simulink model "comm_test_server_OA"  (R2014a)
settings: Solver=ode4  StartTime=0.0  StopTime=inf  FixedStep=0.01  RelTol=1e-3
libraries: SimulinkExecutionControl x1
settings Model: Creator=Tulga Ersal  LastModifiedBy=zhengys
settings OptimizationCC: ExpressionDepthLimit=2147483647
settings DebuggingCC: UnderspecifiedInitializationDetection=Classic  StateNameClashWarn=warning

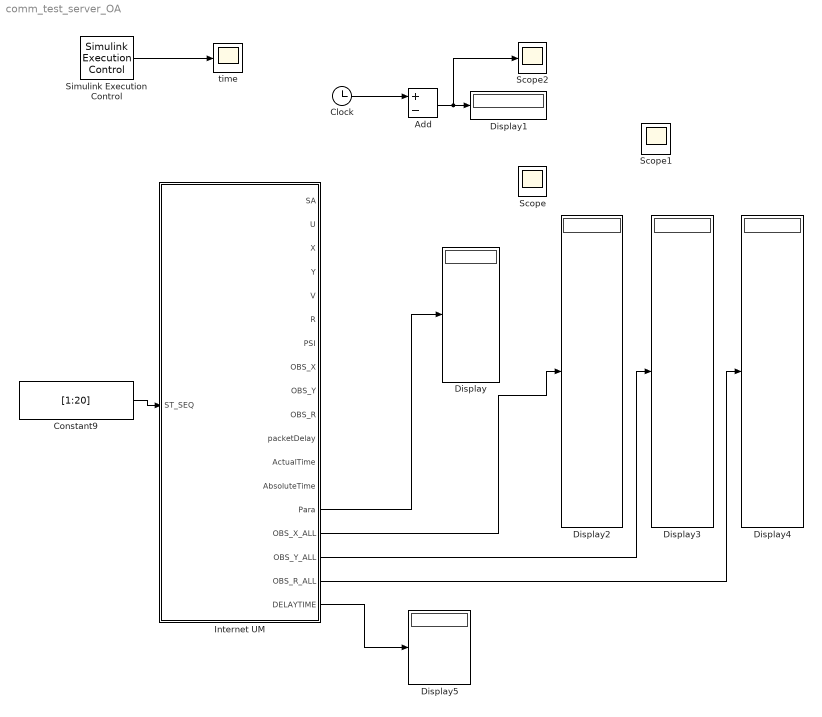
== system comm_test_server_OA ==
  Add : Sum  Inputs=+-
  Clock : Clock
  Constant9 : Constant  Value=[1:20]
  Display{,1..5} (6 alike) : Display
  Internet UM : Subsystem
  Scope : Scope
  Scope1 : Scope
  Scope2 : Scope
      settings: YMin=-0.12  YMax=0.05  SaveName=ScopeData2
  Simulink Execution Control : SimulinkExecutionControl/Simulink Execution Control  proc_pri=REALTIME_PRIORITY_CLASS  thread_pri=THREAD_PRIORITY_TIME_CRITICAL  rt_sim=on  factor=1  ovrrun=Continue execution  Ts=-1
  time : Scope
      settings: TickLabels=on  YMin=1.375  YMax=1.4075  SaveName=ScopeData4
  wires:
  Clock/1 -> Add/1
  Add/1 -> Scope2/1, Display1/1
  Constant9/1 -> Internet UM/1(ST_SEQ)
  Simulink Execution Control/1 -> time/1
  Internet UM/14(Para) -> Display/1
  Internet UM/15(OBS_X_ALL) -> Display2/1
  Internet UM/16(OBS_Y_ALL) -> Display3/1
  Internet UM/17(OBS_R_ALL) -> Display4/1
  Internet UM/18(DELAYTIME) -> Display5/1

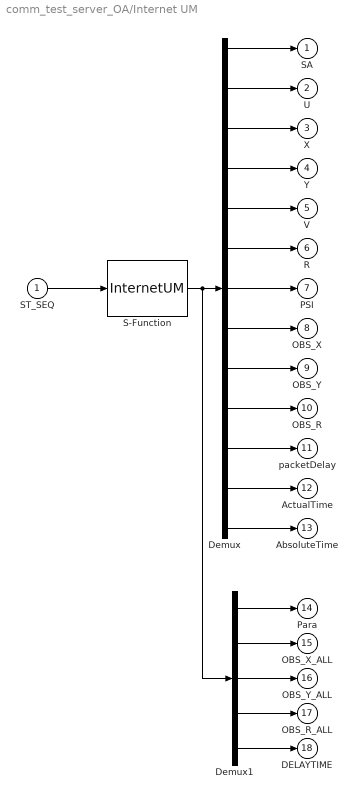
== system comm_test_server_OA/Internet UM ==
  ST_SEQ : Inport
  Demux : Demux  Outputs=[1 1 1 1 1 1 1 3 3 3 1 1 1]
  Demux1 : Demux  Outputs=[7 3 3 3 3]
  S-Function : S-Function  FunctionName=InternetUM  EnableBusSupport=off
  SA : Outport
  U : Outport  Port=2
  X : Outport  Port=3
  Y : Outport  Port=4
  V : Outport  Port=5
  R : Outport  Port=6
  PSI : Outport  Port=7
  OBS_X : Outport  Port=8
  OBS_Y : Outport  Port=9
  OBS_R : Outport  Port=10
  packetDelay : Outport  Port=11
  ActualTime : Outport  Port=12
  AbsoluteTime : Outport  Port=13
  Para : Outport  Port=14
  OBS_X_ALL : Outport  Port=15
  OBS_Y_ALL : Outport  Port=16
  OBS_R_ALL : Outport  Port=17
  DELAYTIME : Outport  Port=18
  wires:
  S-Function/1 -> Demux1/1, Demux/1
  ST_SEQ/1 -> S-Function/1
  Demux/13 -> AbsoluteTime/1
  Demux/11 -> packetDelay/1
  Demux/12 -> ActualTime/1
  Demux/1 -> SA/1
  Demux/2 -> U/1
  Demux/3 -> X/1
  Demux/4 -> Y/1
  Demux/5 -> V/1
  Demux/6 -> R/1
  Demux/7 -> PSI/1
  Demux/8 -> OBS_X/1
  Demux/9 -> OBS_Y/1
  Demux/10 -> OBS_R/1
  Demux1/2 -> OBS_X_ALL/1
  Demux1/1 -> Para/1
  Demux1/3 -> OBS_Y_ALL/1
  Demux1/4 -> OBS_R_ALL/1
  Demux1/5 -> DELAYTIME/1
